simulink model "BatteryController"  (R2025a)
settings: Solver=ode23s  StartTime=0.0  StopTime=10  FixedStep=5e-6  MaxStep=50e-6  RelTol=1e-4  EnableMultiTasking=on
model workspace (MAT data in the model file):
  Fs = 10000
  Fsw = 10000
undefined symbols (not defined in the file or in its folder): Ion, Lithium
libraries: spsSeriesRLCBranchLib x3, slpidlib x3, spsIGBTDiodeLib x2, powerlib_extras x2, spsMultimeterLib x2, spsBatteryLib x1, simulink x1, spsCurrentMeasurementLib x1, spsIdealSwitchLib x1, spsDCVoltageSourceLib x1, spspowerguiLib x1
settings Model: Creator=DELL  LastModifiedBy=mac
settings SolverCC: AlgebraicLoopSolver=TrustRegion
settings DataIOCC: LimitDataPoints=on  SaveFormat=Array  SignalLoggingSaveFormat=ModelDataLogs  ReturnWorkspaceOutputs=off
settings OptimizationCC: ExpressionDepthLimit=2147483647.0  LifeSpan=inf
settings DebuggingCC: UnderspecifiedInitializationDetection=Classic  MergeDetectMultiDrivingBlocksExec=none  SolverPrmCheckMsg=warning  FcnCallInpInsideContextMsg=warning  UnconnectedInputMsg=warning  UnconnectedOutputMsg=warning  UnconnectedLineMsg=warning  StateNameClashWarn=warning  SFUnexpectedBacktrackingDiag=warning  SFNoUnconditionalDefaultTransitionDiag=warning  SFExecutionAtInitializationDiag=none  ArithmeticOperatorsInVariantConditions=warning
settings HardwareCC: ProdBitPerPointer=32.0  ProdBitPerSizeT=32.0  ProdBitPerPtrDiffT=32.0  ProdLargestAtomicFloat=None  ProdIntDivRoundTo=Undefined  ProdEndianess=Unspecified  ProdWordSize=32.0  ProdHWDeviceType=32-bit Generic
settings ModelReferenceCC: EnableRefExpFcnMdlSchedulingChecks=on  PropagateSignalLabelsOutOfModel=off
settings SFSimCC: SimUseLocalCustomCode=off  CustomCodeUndefinedFunction=UseInterfaceOnly
settings RTWCC: RTWUseLocalCustomCode=off  GPUComputeCapability=3.5
settings CodeAppCC: StateflowObjectComments=on
settings GRTTargetCC: TargetLangStandard=C89/C90 (ANSI)  CombineOutputUpdateFcns=off  GRTInterface=on
settings ConfigComp: CovMetricSettings=dw  CovSaveCumulativeToWorkspaceVar=on  CovSaveSingleToWorkspaceVar=on  CovExternalEMLEnable=off  CovSFcnEnable=off
settings SimscapeCC: SimscapeNormalizeSystem=off

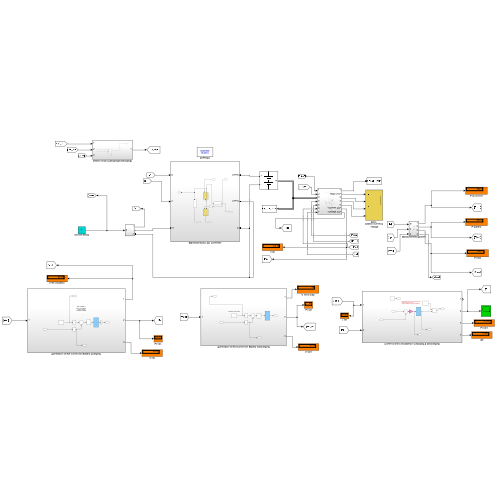
[thumbnail: Simulink's stored preview of the top-level diagram]
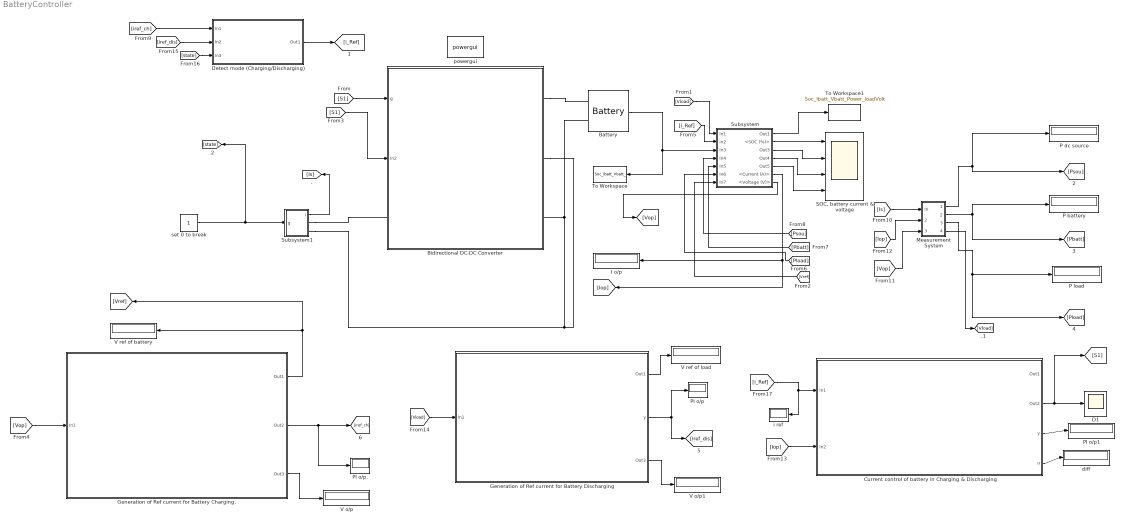
== system BatteryController ==
  "   D1" : Scope
      settings: TimeSpan=0.01960030745580332  ActiveDisplayYMinimum=-0.125  ActiveDisplayYMaximum=1.125  DataLoggingVariableName=VVI  DataLoggingSaveFormat=Array
  Battery : spsBatteryLib/Battery  BatType=Lithium-Ion  NomV=24  NomQ=50  SOC=45  Batt_Tr=1  PresetModel=off  MaxQ=50  MinV=18  FullV=27.9357  Dis_rate=21.7391  R=0.0048  Normal_OP=45.2174  expZone="[25.9293      2.45652]"
      settings: LibrarySourceBlock=electricdrivelib/Extra Sources/Battery
  Bidirectional DC-DC Converter : Subsystem
  Current control of battery in Charging & Discharging : Subsystem
  Detect mode (Charging/Discharging) : Subsystem
  Generation of Ref current for Battery Charging. : Subsystem
  Generation of Ref current for Battery Discharging : Subsystem
  I o/p : Display
  Measurement System : Subsystem
  P battery : Display
  P dc source : Display
  P load : Display
  PI o/p : Display
  PI o/p. : Display
  PI o/p1 : Display
  "SOC, battery current & voltage" : Scope  NumInputPorts=4
      settings: SampleTime=1/Fs  ActiveDisplayYMinimum=46.623431864713254  ActiveDisplayYMaximum=46.866915196882822  DataLoggingVariableName=Soc_Ibatt_Vbatt
  Subsystem : Subsystem
  Subsystem1 : Subsystem
  To Workspace : ToWorkspace  VariableName=Soc_Ibatt_Vbatt_  SampleTime=-1
  To Workspace1 : ToWorkspace  VariableName=Soc_Ibatt_Vbatt_Power_loadVolt  SampleTime=-1
  V o/p : Display
  V o/p1 : Display
  "V ref of battery " : Display
  V ref of load : Display
  diff : Display
  i ref : Display
  powergui : spspowerguiLib/powergui  Priority=1  SimulationMode=Discrete  SampleTime=1e-5  frequency=60  Iterations=50  frequencyindice=0  Pbase=100e6  ErrMax=1e-4  UnitsV=kV  UnitsW=MW  buscounter=0  FunctionMessages=off  echomessages=off  EnableUseOfTLC=off  CurrentSourceSwitches=off  DisableSnubberDevices=off  DisableRonSwitches=off  DisableVfSwitches=off  DisplayEquations=off  AutomaticDiscreteSolvers=off  SolverType=Tustin/Backward Euler (TBE)  Interpol=off  ExternalGateDelay=off  methode=off  Ts=0  x0status=blocks  SPID=off  SwTol=0  HookPort=off  NonlinearTolerance=1e-4  nMaxIteration=100  ContinueOnMaxIteration=off  RestoreLinks=warning  ResistiveCurrentMeasurement=off  Frange=[0:2:500]  Ylog=off  Xlog=on  ShowGrid=off  save=off  variable=ZData  structure=0  ZoomFFT=off  StartTime=0.0  cycles=1  DisplayStyle=1  fundamental=60  FreqAxis=off  MaxFrequency=1000  frequencyindicesteady=1  RmsSteady=1  display=off
  set 0 to break : Constant
  wires:
  Battery/1 -> Subsystem/3(In3), To Workspace/1
  [i_Ref] -> i ref/1, Current control of battery in Charging & Discharging/1(In1)
  set 0 to break/1 -> [state], Subsystem1/1(g)
  Measurement System/2(Out2) -> [Pbatt], P battery/1
  Measurement System/1(Out1) -> [Psou], P dc source/1
  Measurement System/3(Out3) -> [Pload], P load/1
  [Is] -> Measurement System/1(In)
  [Iop] -> Measurement System/2(In1)
  [Vop] -> Measurement System/3(In3)
  Measurement System/4(Out4) -> [Vload]
  [S1] -> Bidirectional DC-DC Converter/1(g)
  [S1] -> Bidirectional DC-DC Converter/2(In2)
  [iref_ch] -> Detect mode (Charging/Discharging)/1(In1)
  [iref_dis] -> Detect mode (Charging/Discharging)/2(In2)
  [state] -> Detect mode (Charging/Discharging)/3(In3)
  Detect mode (Charging/Discharging)/1(Out1) -> [i_Ref]
  Subsystem1/1(i) -> [Is]
  Subsystem/6(<Current (A)>) -> I o/p/1, [Iop]
  [Vload] -> Subsystem/1(In1)
  [i_Ref] -> Subsystem/2(In2)
  [Psou] -> Subsystem/4(In4)
  [Pbatt] -> Subsystem/5(In5)
  [Pload] -> Subsystem/6(In6)
  [Vref] -> Subsystem/7(In7)
  Subsystem/1(Out1) -> To Workspace1/1
  Subsystem/2(<SOC (%)>) -> "SOC, battery current & voltage"/1
  Subsystem/3(Out3) -> "SOC, battery current & voltage"/2
  Subsystem/4(Out4) -> "SOC, battery current & voltage"/3
  Subsystem/5(Out5) -> "SOC, battery current & voltage"/4
  Subsystem/7(<Voltage (V)>) -> [Vop]
  Generation of Ref current for Battery Charging./2(Out2) -> PI o/p./1, [iref_ch]
  Generation of Ref current for Battery Charging./1(Out1) -> [Vref], "V ref of battery "/1
  [Vop] -> Generation of Ref current for Battery Charging./1(In1)
  Generation of Ref current for Battery Charging./3(Out3) -> V o/p/1
  Generation of Ref current for Battery Discharging/2(y) -> [iref_dis], PI o/p/1
  [Vload] -> Generation of Ref current for Battery Discharging/1(In1)
  Generation of Ref current for Battery Discharging/1(Out1) -> V ref of load/1
  Generation of Ref current for Battery Discharging/3(Out3) -> V o/p1/1
  Current control of battery in Charging & Discharging/2(Out2) -> [S1], "   D1"/1
  [Iop] -> Current control of battery in Charging & Discharging/2(In2)
  Current control of battery in Charging & Discharging/3(y) -> PI o/p1/1
  Current control of battery in Charging & Discharging/4(u) -> diff/1
  connections:
  Bidirectional DC-DC Converter/RConn2 -- Subsystem1/RConn2 -- Battery/LConn2 -- Bidirectional DC-DC Converter/RConn3
  Bidirectional DC-DC Converter/RConn1 -- Battery/LConn1
  Subsystem1/RConn1 -- Bidirectional DC-DC Converter/LConn1

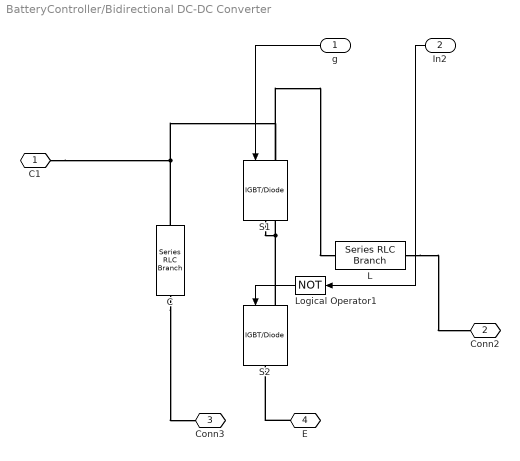
== system BatteryController/Bidirectional DC-DC Converter ==
  g : Inport
  In2 : Inport  Port=2
  C : spsSeriesRLCBranchLib/Series RLC Branch  LConnTagsString=__new0  RConnTagsString=__new0  BranchType=RC  Resistance=0.003  Inductance=1.25e-6  SetiL0=on  InitialCurrent=0  Capacitance=1000e-6  Setx0=off  InitialVoltage=0  Measurements=Branch voltage and current
  L : spsSeriesRLCBranchLib/Series RLC Branch  LConnTagsString=__new0  RConnTagsString=__new0  BranchType=RL  Resistance=0.05  Inductance=5.76e-4  SetiL0=on  InitialCurrent=0  Capacitance=1e-6  Setx0=off  InitialVoltage=0  Measurements=Branch voltage and current
  Logical Operator1 : Logic  Operator=NOT  AllPortsSameDT=off  OutDataTypeStr=boolean
  S1 : spsIGBTDiodeLib/IGBT//Diode  Ron=0.004  Rs=1e5  Cs=inf  Measurements=off
  S2 : spsIGBTDiodeLib/IGBT//Diode  Ron=0.004  Rs=1e5  Cs=inf  Measurements=off
  C1 : PMIOPort  Side=Left
  Conn2 : PMIOPort  Port=2  Side=Right
  Conn3 : PMIOPort  Port=3  Side=Right
  E : PMIOPort  Port=4  Side=Right
  wires:
  In2/1 -> Logical Operator1/1
  Logical Operator1/1 -> S2/1
  g/1 -> S1/1
  connections:
  E/RConn1 -- S2/RConn1
  L/RConn1 -- Conn2/RConn1
  C/RConn1 -- Conn3/RConn1
  C/LConn1 -- C1/RConn1 -- S1/LConn1
  S2/LConn1 -- S1/RConn1 -- L/LConn1

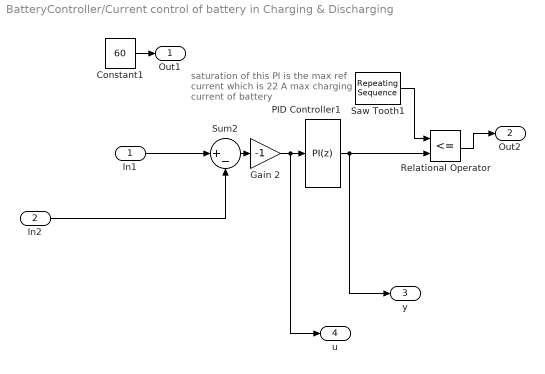
== system BatteryController/Current control of battery in Charging & Discharging ==
  note: saturation of this PI is the max ref
      | current which is 22 A
      | max charging current of battery
  In1 : Inport
  In2 : Inport  Port=2
  Constant1 : Constant  Value=60
  Gain 2 : Gain  Gain=-1
  PID Controller1 : slpidlib/PID Controller  Controller=PI  Form=Parallel  TimeDomain=Discrete-time  UseExternalTs=off  SampleTime=5e-6  IntegratorMethod=Forward Euler  FilterMethod=Forward Euler  ControllerParametersSource=internal  P=0.05  I=10  UseKiTs=off  D=0.5  UseExternalDerivativeSource=off  N=100  UseFilter=on  TunerSelectOption=Transfer Function Based (PID Tuner App)  InitialConditionSource=internal  InitialConditionForIntegrator=0  InitialConditionForFilter=0  DifferentiatorICPrevScaledInput=0  ExternalReset=none  TrackingMode=off  Kt=1  LimitOutput=on  SatLimitsSource=internal  UpperSaturationLimit=0.95  LowerSaturationLimit=0  LinearizeAsGain=on  AntiWindupMode=none  Kb=1  LimitIntegrator=off  UpperIntegratorSaturationLimit=inf  LowerIntegratorSaturationLimit=-inf  POutMin=[]  POutMax=[]  IOutMin=[]  IOutMax=[]  DOutMin=[]  DOutMax=[]  NOutMin=[]  NOutMax=[]  SumOutMin=[]  SumOutMax=[]  SaturationOutMin=[]  SaturationOutMax=[]  PParamMin=[]  PParamMax=[]  IParamMin=[]  IParamMax=[]  DParamMin=[]  DParamMax=[]  NParamMin=[]  NParamMax=[]  KbParamMin=[]  KbParamMax=[]  KtParamMin=[]  KtParamMax=[]  KbOutMin=[]  KbOutMax=[]  KtOutMin=[]  KtOutMax=[]  IntegratorOutMin=[]  IntegratorOutMax=[]  FilterOutMin=[]  FilterOutMax=[]  SumI1OutMin=[]  SumI1OutMax=[]  SumI2OutMin=[]  SumI2OutMax=[]  SumI3OutMin=[]  SumI3OutMax=[]  SumI4OutMin=[]  SumI4OutMax=[]  SumDOutMin=[]  SumDOutMax=[]  DifferentiatorOutMin=[]  DifferentiatorOutMax=[]  FilterDiffOutCoefMin=[]  FilterDiffOutCoefMax=[]  ReciprocalOutMin=[]  ReciprocalOutMax=[]  SumDenOutMin=[]  SumDenOutMax=[]  SumNumOutMin=[]  SumNumOutMax=[]  DivideOutMin=[]  DivideOutMax=[]  UdiffTsProdOutMin=[]  UdiffTsProdOutMax=[]  NTsProdOutMin=[]  NTsProdOutMax=[]  UintegralTsProdOutMin=[]  UintegralTsProdOutMax=[]  UngainTsProdOutMin=[]  UngainTsProdOutMax=[]  ClampingZeroOutDataTypeStr=Inherit: Inherit via back propagation  ClampingZeroOutMin=[]  ClampingZeroOutMax=[]  FilterDenConstantOutDataTypeStr=Inherit: Inherit via back propagation  FilterDenConstantOutMin=[]  FilterDenConstantOutMax=[]  PCopyOutDataTypeStr=Inherit: Inherit via back propagation  PCopyOutMin=[]  PCopyOutMax=[]  NCopyOutDataTypeStr=Inherit: Inherit via back propagation  NCopyOutMin=[]  NCopyOutMax=[]  IntegratorContinuousStateAttributes=''  IntegratorStateMustResolveToSignalObject=off  IntegratorRTWStateStorageClass=Auto  FilterContinuousStateAttributes=''  FilterStateMustResolveToSignalObject=off  FilterRTWStateStorageClass=Auto  ParallelPVariant=InternalParameters  IdealPVariant=Disabled  IVariant=InternalParameters  DVariant=Disabled  IntegratorVariant=Discrete  SatVariant=Enabled  AWVariant=Passthrough  PCopyVariant=Disabled  TRVariant=Disabled  FdbkBlocksVariant=Forward  IdealPFdbkVariant=Disabled  SatFdbkVariant=Disabled  DerivativeFilterVariant=Disabled  NVariant=Disabled  NCopyVariant=Disabled_SignalSpec  FilterICVariant=Disabled  IntegratorICVariant=InternalICs  ExternalResetVariant=Disabled  TRSumVariant=Passthrough  SumFdbkVariant=Disabled  SumVariant=Sum_PI  TsampFilterVariant=InternalTs  TsampNgainVariant=Passthrough  TsampIntegralVariant=Disabled_SignalSpec  ExternalSaturationOutDataTypeStr=Inherit: Same as second input  DerivativeSourceVariant=Disabled  PreIntVariant=InternalPreInt
  Relational Operator : RelationalOperator  Operator=<=  OutDataTypeStr=boolean  RndMeth=Simplest  InputSameDT=off
  Saw Tooth1 : simulink/Sources/Repeating Sequence  rep_seq_t="[0     1/Fsw ]"  rep_seq_y="[0 1  ]"
  Sum2 : Sum  Inputs=|+-
  Out1 : Outport
  Out2 : Outport  Port=2
  y : Outport  Port=3
  u : Outport  Port=4
  wires:
  Constant1/1 -> Out1/1
  In2/1 -> Sum2/2
  In1/1 -> Sum2/1
  Relational Operator/1 -> Out2/1
  Saw Tooth1/1 -> Relational Operator/1
  Gain 2/1 -> u/1, PID Controller1/1
  Sum2/1 -> Gain 2/1
  PID Controller1/1 -> y/1, Relational Operator/2

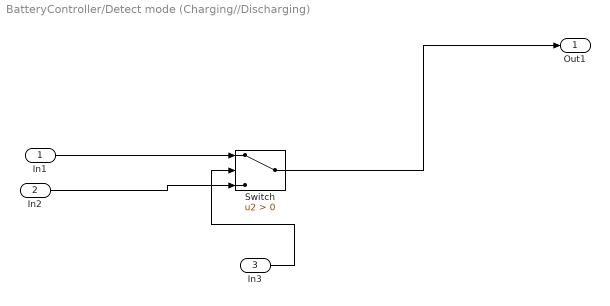
== system BatteryController/Detect mode (Charging//Discharging) ==
  In1 : Inport
  In2 : Inport  Port=2
  In3 : Inport  Port=3
  Switch : Switch  Criteria=u2 > Threshold  SaturateOnIntegerOverflow=off  InputSameDT=off
  Out1 : Outport
  wires:
  In2/1 -> Switch/3
  In1/1 -> Switch/1
  In3/1 -> Switch/2
  Switch/1 -> Out1/1

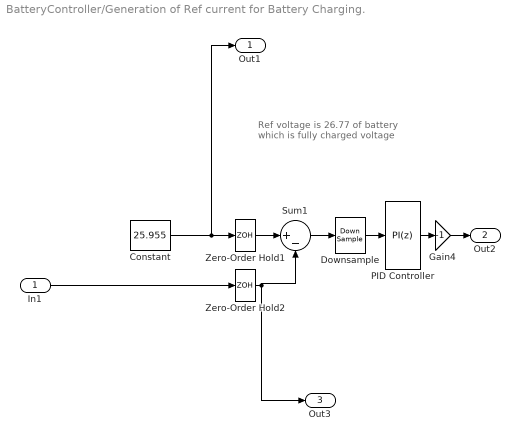
== system BatteryController/Generation of Ref current for Battery Charging. ==
  note: Ref voltage is 26.77 of battery
      | which is fully charged voltage
  In1 : Inport
  Constant : Constant  Value=25.955
  Downsample : DownSample  N=Fs/Fsw  InputProcessing=Inherited (this choice will be removed - see release notes)  RateOptions=Allow multirate processing
  Gain4 : Gain  Gain=-1
  PID Controller : slpidlib/PID Controller  Controller=PI  Form=Parallel  TimeDomain=Discrete-time  UseExternalTs=off  SampleTime=1/Fsw  IntegratorMethod=Forward Euler  FilterMethod=Forward Euler  ControllerParametersSource=internal  P=50  I=1000  UseKiTs=off  D=0.5  UseExternalDerivativeSource=off  N=100  UseFilter=on  TunerSelectOption=Transfer Function Based (PID Tuner App)  InitialConditionSource=internal  InitialConditionForIntegrator=0  InitialConditionForFilter=0  DifferentiatorICPrevScaledInput=0  ExternalReset=none  TrackingMode=off  Kt=1  LimitOutput=on  SatLimitsSource=internal  UpperSaturationLimit=22  LowerSaturationLimit=0  LinearizeAsGain=on  AntiWindupMode=none  Kb=1  LimitIntegrator=off  UpperIntegratorSaturationLimit=inf  LowerIntegratorSaturationLimit=-inf  POutMin=[]  POutMax=[]  IOutMin=[]  IOutMax=[]  DOutMin=[]  DOutMax=[]  NOutMin=[]  NOutMax=[]  SumOutMin=[]  SumOutMax=[]  SaturationOutMin=[]  SaturationOutMax=[]  PParamMin=[]  PParamMax=[]  IParamMin=[]  IParamMax=[]  DParamMin=[]  DParamMax=[]  NParamMin=[]  NParamMax=[]  KbParamMin=[]  KbParamMax=[]  KtParamMin=[]  KtParamMax=[]  KbOutMin=[]  KbOutMax=[]  KtOutMin=[]  KtOutMax=[]  IntegratorOutMin=[]  IntegratorOutMax=[]  FilterOutMin=[]  FilterOutMax=[]  SumI1OutMin=[]  SumI1OutMax=[]  SumI2OutMin=[]  SumI2OutMax=[]  SumI3OutMin=[]  SumI3OutMax=[]  SumI4OutMin=[]  SumI4OutMax=[]  SumDOutMin=[]  SumDOutMax=[]  DifferentiatorOutMin=[]  DifferentiatorOutMax=[]  FilterDiffOutCoefMin=[]  FilterDiffOutCoefMax=[]  ReciprocalOutMin=[]  ReciprocalOutMax=[]  SumDenOutMin=[]  SumDenOutMax=[]  SumNumOutMin=[]  SumNumOutMax=[]  DivideOutMin=[]  DivideOutMax=[]  UdiffTsProdOutMin=[]  UdiffTsProdOutMax=[]  NTsProdOutMin=[]  NTsProdOutMax=[]  UintegralTsProdOutMin=[]  UintegralTsProdOutMax=[]  UngainTsProdOutMin=[]  UngainTsProdOutMax=[]  ClampingZeroOutDataTypeStr=Inherit: Inherit via back propagation  ClampingZeroOutMin=[]  ClampingZeroOutMax=[]  FilterDenConstantOutDataTypeStr=Inherit: Inherit via back propagation  FilterDenConstantOutMin=[]  FilterDenConstantOutMax=[]  PCopyOutDataTypeStr=Inherit: Inherit via back propagation  PCopyOutMin=[]  PCopyOutMax=[]  NCopyOutDataTypeStr=Inherit: Inherit via back propagation  NCopyOutMin=[]  NCopyOutMax=[]  IntegratorContinuousStateAttributes=''  IntegratorStateMustResolveToSignalObject=off  IntegratorRTWStateStorageClass=Auto  FilterContinuousStateAttributes=''  FilterStateMustResolveToSignalObject=off  FilterRTWStateStorageClass=Auto  ParallelPVariant=InternalParameters  IdealPVariant=Disabled  IVariant=InternalParameters  DVariant=Disabled  IntegratorVariant=Discrete  SatVariant=Enabled  AWVariant=Passthrough  PCopyVariant=Disabled  TRVariant=Disabled  FdbkBlocksVariant=Forward  IdealPFdbkVariant=Disabled  SatFdbkVariant=Disabled  DerivativeFilterVariant=Disabled  NVariant=Disabled  NCopyVariant=Disabled_SignalSpec  FilterICVariant=Disabled  IntegratorICVariant=InternalICs  ExternalResetVariant=Disabled  TRSumVariant=Passthrough  SumFdbkVariant=Disabled  SumVariant=Sum_PI  TsampFilterVariant=InternalTs  TsampNgainVariant=Passthrough  TsampIntegralVariant=Disabled_SignalSpec  ExternalSaturationOutDataTypeStr=Inherit: Same as second input  DerivativeSourceVariant=Disabled  PreIntVariant=InternalPreInt
  Sum1 : Sum  Inputs=|+-
  Zero-Order Hold1 : ZeroOrderHold  SampleTime=1/Fs
  Zero-Order Hold2 : ZeroOrderHold  SampleTime=1/Fs
  Out1 : Outport
  Out2 : Outport  Port=2
  Out3 : Outport  Port=3
  wires:
  Gain4/1 -> Out2/1
  Zero-Order Hold1/1 -> Sum1/1
  PID Controller/1 -> Gain4/1
  In1/1 -> Zero-Order Hold2/1
  Constant/1 -> Out1/1, Zero-Order Hold1/1
  Downsample/1 -> PID Controller/1
  Sum1/1 -> Downsample/1
  Zero-Order Hold2/1 -> Out3/1, Sum1/2

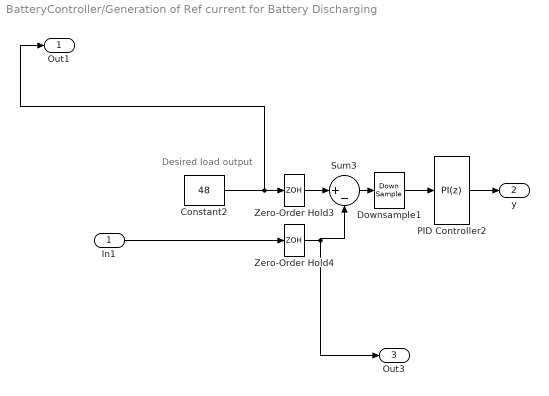
== system BatteryController/Generation of Ref current for Battery Discharging ==
  note: Desired load output
  In1 : Inport
  Constant2 : Constant  Value=48
  Downsample1 : DownSample  N=Fs/Fsw  InputProcessing=Inherited (this choice will be removed - see release notes)  RateOptions=Allow multirate processing
  PID Controller2 : slpidlib/PID Controller  Controller=PI  Form=Parallel  TimeDomain=Discrete-time  UseExternalTs=off  SampleTime=1/Fsw  IntegratorMethod=Forward Euler  FilterMethod=Forward Euler  ControllerParametersSource=internal  P=0.5  I=50  UseKiTs=off  D=0.5  UseExternalDerivativeSource=off  N=100  UseFilter=on  TunerSelectOption=Transfer Function Based (PID Tuner App)  InitialConditionSource=internal  InitialConditionForIntegrator=0  InitialConditionForFilter=0  DifferentiatorICPrevScaledInput=0  ExternalReset=none  TrackingMode=off  Kt=1  LimitOutput=on  SatLimitsSource=internal  UpperSaturationLimit=22  LowerSaturationLimit=0  LinearizeAsGain=on  AntiWindupMode=none  Kb=1  LimitIntegrator=off  UpperIntegratorSaturationLimit=inf  LowerIntegratorSaturationLimit=-inf  POutMin=[]  POutMax=[]  IOutMin=[]  IOutMax=[]  DOutMin=[]  DOutMax=[]  NOutMin=[]  NOutMax=[]  SumOutMin=[]  SumOutMax=[]  SaturationOutMin=[]  SaturationOutMax=[]  PParamMin=[]  PParamMax=[]  IParamMin=[]  IParamMax=[]  DParamMin=[]  DParamMax=[]  NParamMin=[]  NParamMax=[]  KbParamMin=[]  KbParamMax=[]  KtParamMin=[]  KtParamMax=[]  KbOutMin=[]  KbOutMax=[]  KtOutMin=[]  KtOutMax=[]  IntegratorOutMin=[]  IntegratorOutMax=[]  FilterOutMin=[]  FilterOutMax=[]  SumI1OutMin=[]  SumI1OutMax=[]  SumI2OutMin=[]  SumI2OutMax=[]  SumI3OutMin=[]  SumI3OutMax=[]  SumI4OutMin=[]  SumI4OutMax=[]  SumDOutMin=[]  SumDOutMax=[]  DifferentiatorOutMin=[]  DifferentiatorOutMax=[]  FilterDiffOutCoefMin=[]  FilterDiffOutCoefMax=[]  ReciprocalOutMin=[]  ReciprocalOutMax=[]  SumDenOutMin=[]  SumDenOutMax=[]  SumNumOutMin=[]  SumNumOutMax=[]  DivideOutMin=[]  DivideOutMax=[]  UdiffTsProdOutMin=[]  UdiffTsProdOutMax=[]  NTsProdOutMin=[]  NTsProdOutMax=[]  UintegralTsProdOutMin=[]  UintegralTsProdOutMax=[]  UngainTsProdOutMin=[]  UngainTsProdOutMax=[]  ClampingZeroOutDataTypeStr=Inherit: Inherit via back propagation  ClampingZeroOutMin=[]  ClampingZeroOutMax=[]  FilterDenConstantOutDataTypeStr=Inherit: Inherit via back propagation  FilterDenConstantOutMin=[]  FilterDenConstantOutMax=[]  PCopyOutDataTypeStr=Inherit: Inherit via back propagation  PCopyOutMin=[]  PCopyOutMax=[]  NCopyOutDataTypeStr=Inherit: Inherit via back propagation  NCopyOutMin=[]  NCopyOutMax=[]  IntegratorContinuousStateAttributes=''  IntegratorStateMustResolveToSignalObject=off  IntegratorRTWStateStorageClass=Auto  FilterContinuousStateAttributes=''  FilterStateMustResolveToSignalObject=off  FilterRTWStateStorageClass=Auto  ParallelPVariant=InternalParameters  IdealPVariant=Disabled  IVariant=InternalParameters  DVariant=Disabled  IntegratorVariant=Discrete  SatVariant=Enabled  AWVariant=Passthrough  PCopyVariant=Disabled  TRVariant=Disabled  FdbkBlocksVariant=Forward  IdealPFdbkVariant=Disabled  SatFdbkVariant=Disabled  DerivativeFilterVariant=Disabled  NVariant=Disabled  NCopyVariant=Disabled_SignalSpec  FilterICVariant=Disabled  IntegratorICVariant=InternalICs  ExternalResetVariant=Disabled  TRSumVariant=Passthrough  SumFdbkVariant=Disabled  SumVariant=Sum_PI  TsampFilterVariant=InternalTs  TsampNgainVariant=Passthrough  TsampIntegralVariant=Disabled_SignalSpec  ExternalSaturationOutDataTypeStr=Inherit: Same as second input  DerivativeSourceVariant=Disabled  PreIntVariant=InternalPreInt
  Sum3 : Sum  Inputs=|+-
  Zero-Order Hold3 : ZeroOrderHold  SampleTime=1/Fs
  Zero-Order Hold4 : ZeroOrderHold  SampleTime=1/Fs
  Out1 : Outport
  y : Outport  Port=2
  Out3 : Outport  Port=3
  wires:
  In1/1 -> Zero-Order Hold4/1
  PID Controller2/1 -> y/1
  Sum3/1 -> Downsample1/1
  Downsample1/1 -> PID Controller2/1
  Zero-Order Hold3/1 -> Sum3/1
  Zero-Order Hold4/1 -> Out3/1, Sum3/2
  Constant2/1 -> Out1/1, Zero-Order Hold3/1

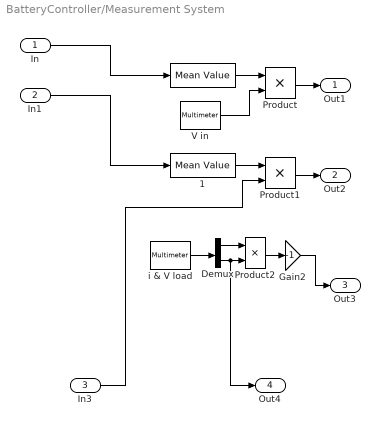
== system BatteryController/Measurement System ==
  In : Inport
  In1 : Inport  Port=2
  In3 : Inport  Port=3
  "   " : powerlib_extras/Measurements/Mean Value  Period=1/Fsw
  "   1" : powerlib_extras/Measurements/Mean Value  Period=1/Fsw
  Demux : Demux  Outputs=2
  Gain2 : Gain  Gain=-1
  Product : Product
  Product1 : Product
  Product2 : Product
  V in : spsMultimeterLib/Multimeter  L=7  sel=4  Gain=1  OutputType=Complex  PlotAtSimulationStop=off  PhasorSimulation=off
  i & V load : spsMultimeterLib/Multimeter  L=7  sel=[7 3]  Gain=[1 1]  OutputType=Complex  PlotAtSimulationStop=off  PhasorSimulation=off
  Out1 : Outport
  Out2 : Outport  Port=2
  Out3 : Outport  Port=3
  Out4 : Outport  Port=4
  wires:
  Product/1 -> Out1/1
  In1/1 -> "   1"/1
  In/1 -> "   "/1
  Product2/1 -> Gain2/1
  Product1/1 -> Out2/1
  Gain2/1 -> Out3/1
  Demux/2 -> Out4/1, Product2/2
  Demux/1 -> Product2/1
  In3/1 -> Product1/2
  "   1"/1 -> Product1/1
  i & V load/1 -> Demux/1
  V in/1 -> Product/2
  "   "/1 -> Product/1

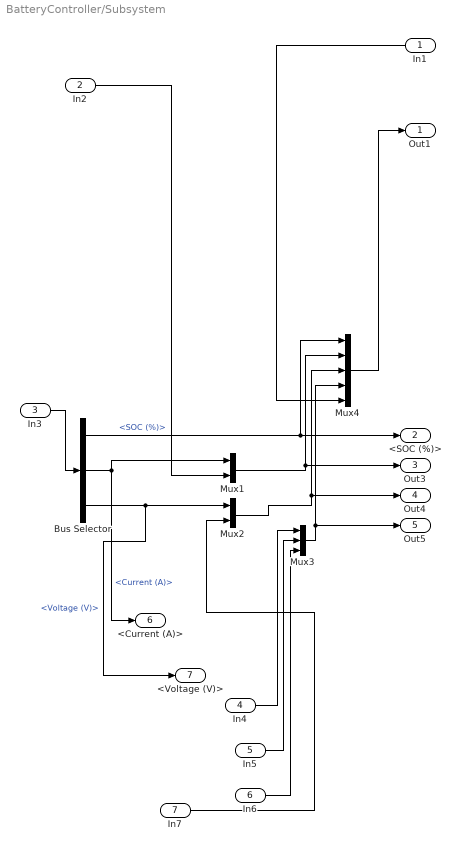
== system BatteryController/Subsystem ==
  In1 : Inport
  In2 : Inport  Port=2
  In3 : Inport  Port=3
  In4 : Inport  Port=4
  In5 : Inport  Port=5
  In6 : Inport  Port=6
  In7 : Inport  Port=7
  Bus Selector : BusSelector  OutputSignals=SOC (%),Current (A),Voltage (V)
  Mux1 : Mux  Inputs=2
  Mux2 : Mux  Inputs=2
  Mux3 : Mux  Inputs=3
  Mux4 : Mux  Inputs=5
  Out1 : Outport
  <SOC (%)> : Outport  Port=2
  Out3 : Outport  Port=3
  Out4 : Outport  Port=4
  Out5 : Outport  Port=5
  <Current (A)> : Outport  Port=6
  <Voltage (V)> : Outport  Port=7
  wires:
  In2/1 -> Mux1/2
  In7/1 -> Mux2/2
  In5/1 -> Mux3/2
  Bus Selector/3 -> <Voltage (V)>/1, Mux2/1  "<Voltage (V)>"
  Mux1/1 -> Out3/1, Mux4/2
  In1/1 -> Mux4/5
  Mux3/1 -> Out5/1, Mux4/4
  In3/1 -> Bus Selector/1
  Bus Selector/2 -> <Current (A)>/1, Mux1/1  "<Current (A)>"
  In4/1 -> Mux3/1
  In6/1 -> Mux3/3
  Mux4/1 -> Out1/1
  Bus Selector/1 -> <SOC (%)>/1, Mux4/1  "<SOC (%)>"
  Mux2/1 -> Out4/1, Mux4/3

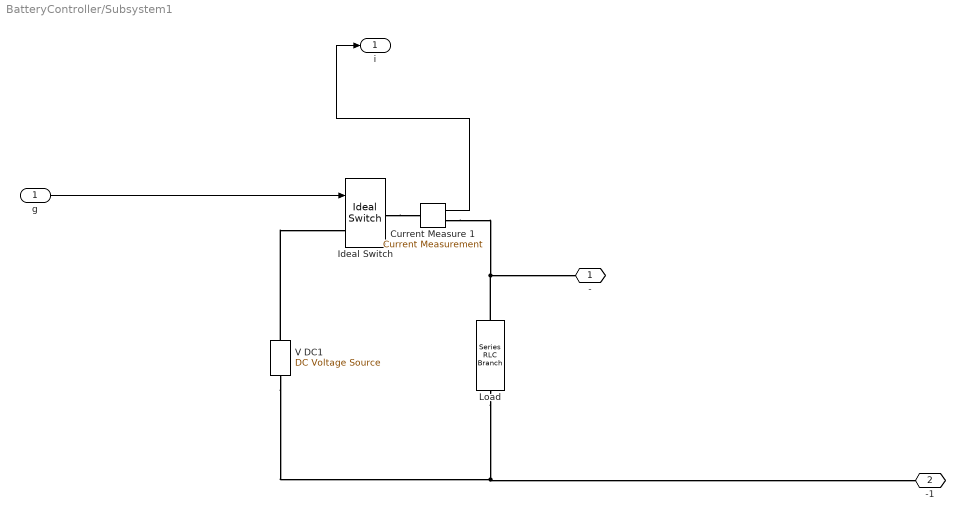
== system BatteryController/Subsystem1 ==
  g : Inport
  Current Measure 1 : spsCurrentMeasurementLib/Current Measurement  PhasorSimulation=off  OutputType=Complex  PSBequivalent=0
  Ideal Switch : spsIdealSwitchLib/Ideal Switch  Ron=0.1  Lon=0  IC=0  Rs=1e5  Cs=inf  Measurements=off
  Load : spsSeriesRLCBranchLib/Series RLC Branch  LConnTagsString=__new0  RConnTagsString=__new0  BranchType=R  Resistance=6  Inductance=1.25e-6  SetiL0=on  InitialCurrent=0  Capacitance=1000e-6  Setx0=off  InitialVoltage=0  Measurements=Branch voltage and current
  V DC1 : spsDCVoltageSourceLib/DC Voltage Source  Amplitude=48  Measurements=Voltage
  - : PMIOPort  Side=Right
  -1 : PMIOPort  Port=2  Side=Right
  i : Outport
  wires:
  Current Measure 1/1 -> i/1
  g/1 -> Ideal Switch/1
  connections:
  V DC1/RConn1 -- Ideal Switch/LConn1
  V DC1/LConn1 -- -1/RConn1 -- Load/RConn1
  Current Measure 1/RConn1 -- -/RConn1 -- Load/LConn1
  Ideal Switch/RConn1 -- Current Measure 1/LConn1
